simulink model "animation_th"  (R2022a)
settings: Solver=VariableStepAuto  StartTime=0.0  StopTime=inf  RelTol=1e-3
libraries: animation_cl x1
settings Model: Creator=mcobb  LastModifiedBy=lhill8
settings SolverCC: AlgebraicLoopSolver=TrustRegion
settings DebuggingCC: UnconnectedInputMsg=warning  UnconnectedOutputMsg=warning  UnconnectedLineMsg=warning  SFMachineParentedDataDiag=warning  ArithmeticOperatorsInVariantConditions=warning
settings SFSimCC: CustomCodeUndefinedFunction=UseInterfaceOnly

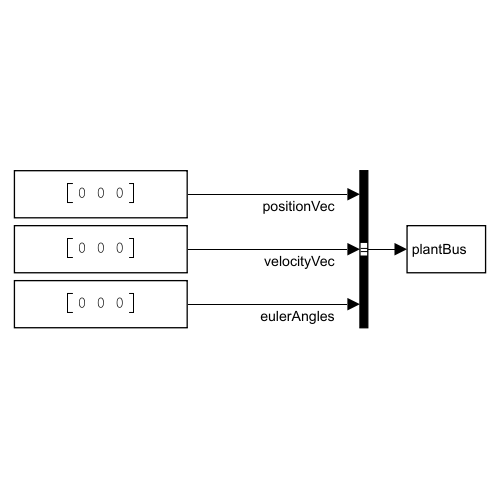
[thumbnail: Simulink's stored preview of the top-level diagram]
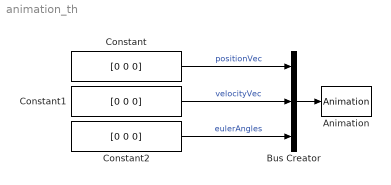
== system animation_th ==
  Animation : animation_cl/Animation  animSampleTime=0.1  scaleFactor=1  elevation=75  radius=400  vidLogEnbl=on  vidDims=[240 480]
  Bus Creator : BusCreator  Inputs=3  OutDataTypeStr=Bus: plantBus  NonVirtualBus=on
      settings: InheritFromInputs=off
  Constant : Constant  Value=[0 0 0]
  Constant1 : Constant  Value=[0 0 0]
  Constant2 : Constant  Value=[0 0 0]
  wires:
  Bus Creator/1 -> Animation/1
  Constant/1 -> Bus Creator/1  "positionVec"
  Constant1/1 -> Bus Creator/2  "velocityVec"
  Constant2/1 -> Bus Creator/3  "eulerAngles"
